simulink model "RI_JB_PI_2"  (R2013b)
settings: Solver=ode45  StartTime=0.0  StopTime=50  MaxStep=tau/10/25  RelTol=1e-3
InitFcn:
  | % Modellparaméterek
  | J = 0.1;
  | B = 0.01;
  | omega_0 = 0;
  | 
  | % Rendszerparaméterek
  | K = 1/B;
  | tau = J/B;
  | 
  | % PI-hangolás ZPK
  | T_I_ZPK = tau;
  | K_PI_ZPK = 1/K * 10;
  | 
  | % PI-hangolás MRZK
  | xi_CL = 1;
  | tau_CL = tau/10;
  | 
  | K_PI_MRZK = (2*xi_CL*tau - tau_CL)/(K*tau_CL);
  | T_I_MRZK = (2*xi_CL*tau - tau_CL)*tau_CL/tau;
libraries: RI_MK x4, simulink x2
settings Model: Creator=Szalay  LastModifiedBy=Szalay

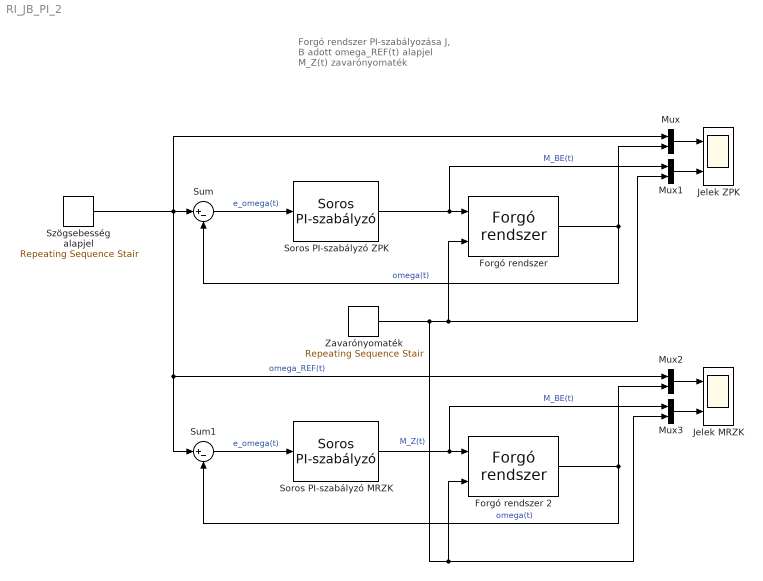
== system RI_JB_PI_2 ==
  note: Forgó rendszer PI-szabályozása
      | J, B adott
      | omega_REF(t) alapjel
      | M_Z(t) zavarónyomaték
  Forgó rendszer : RI_MK/Forgó rendszer  J=J  B=B  omega_0=omega_0
  Forgó rendszer 2 : RI_MK/Forgó rendszer  J=J  B=B  omega_0=omega_0
  Jelek MRZK : Scope  NumInputPorts=2
      settings: ShowLegends=on  YMin=-5~-5  YMax=5~5
  Jelek ZPK : Scope  NumInputPorts=2
      settings: ShowLegends=on  YMin=-5~-5  YMax=5~5
  Mux{,1..3} (4 alike) : Mux  Inputs=2
  Soros PI-szabályzó MRZK : RI_MK/Soros PI-szabályzó  K_PI=K_PI_MRZK  T_I=T_I_MRZK
  Soros PI-szabályzó ZPK : RI_MK/Soros PI-szabályzó  K_PI=K_PI_ZPK  T_I=T_I_ZPK
  Sum : Sum  Inputs=|+-
  Sum1 : Sum  Inputs=|+-
  Szögsebesség alapjel : simulink/Sources/Repeating Sequence Stair  OutValues=[3, -2]  tsamp=25  OutMin=[]  OutMax=[]  OutDataTypeStr=double  OutputDataTypeScalingMode=double  OutDataType=fixdt(0,8)  ConRadixGroup=Best Precision: Vector-wise  OutScaling=2^-12
  Zavarónyomaték : simulink/Sources/Repeating Sequence Stair  OutValues=[0, -2]/10  tsamp=30  OutMin=[]  OutMax=[]  OutDataTypeStr=double  OutputDataTypeScalingMode=double  OutDataType=fixdt(0,8)  ConRadixGroup=Best Precision: Vector-wise  OutScaling=2^-12
  wires:
  Soros PI-szabályzó ZPK/1 -> Mux1/1, Forgó rendszer/1  "M_BE(t)"
  Sum/1 -> Soros PI-szabályzó ZPK/1  "e_omega(t)"
  Forgó rendszer/1 -> Sum/2, Mux/2  "omega(t)"
  Mux/1 -> Jelek ZPK/1
  Mux1/1 -> Jelek ZPK/2
  Soros PI-szabályzó MRZK/1 -> Mux3/1, Forgó rendszer 2/1  "M_BE(t)"
  Sum1/1 -> Soros PI-szabályzó MRZK/1  "e_omega(t)"
  Forgó rendszer 2/1 -> Sum1/2, Mux2/2  "omega(t)"
  Szögsebesség alapjel/1 -> Sum1/1, Mux2/1, Mux/1, Sum/1  "omega_REF(t)"
  Mux2/1 -> Jelek MRZK/1
  Zavarónyomaték/1 -> Forgó rendszer 2/2, Mux3/2, Forgó rendszer/2, Mux1/2  "M_Z(t)"
  Mux3/1 -> Jelek MRZK/2
